simulink model "template_2018b_D"  (R2020a)
settings: Solver=ode1  StartTime=0.0  StopTime=2  FixedStep=1e-6  RelTol=1e-3
undefined symbols (not defined in the file or in its folder): Ion, Lithium
libraries: powerlib x13, powerlib_meascontrol x2, electricdrivelib x1, re_lib x1
settings Model: Creator=ander  LastModifiedBy=delfi
settings DebuggingCC: SFMachineParentedDataDiag=error  ArithmeticOperatorsInVariantConditions=warning
settings SFSimCC: CustomCodeUndefinedFunction=UseInterfaceOnly

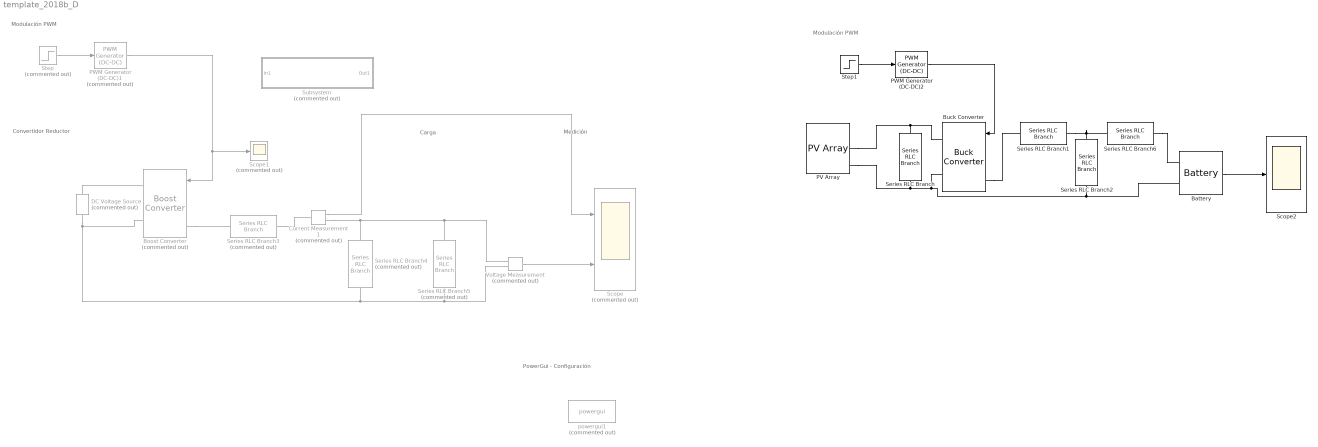
== system template_2018b_D ==
  note: Medición
  note: PowerGui - Configuración
  note: Carga
  note: Convertidor Reductor
  note: Modulación PWM
  note: Modulación PWM
  Battery : electricdrivelib/Extra Sources/Battery  BatType=Lithium-Ion  ShowTempParam=off  ThermalPreset=no  ShowAgeParam=off  NomV=7.2  NomQ=5.4  SOC=100  Batt_Tr=30  PresetModel=on  MaxQ=5.4  MinV=5.4  FullV=8.3807  Dis_rate=2.3478  R=0.013333  Normal_OP=4.8835  expZone="[7.7788      0.2653]"  current=[6.5 13 32.5]  Units=Time  Tci=20  NomT=20  T2=-30  MaxQ2=4.8  FullV2=7.1  Normal_OP2=5.655  expZone2="[6.58           1]"  Rca=0.6  ti=2000  Dp=0  Neq0=0  Tsim=1e6  Ta1=25  Qeol=5.4*0.9  Reol=0.013333*1.2  Char_age=[2.3478, 3]  Dis_age=[2.3478, 10]  N1=1500  N2=10500  N3=1000  N4=1400  Ta2=45  N5=950
  Boost Converter : powerlib/Power Electronics/Boost Converter  Commented=on  ModelType=Switching devices  Ron=1e-3  Rs=1e6  Cs=inf  Vforward=[0,0]  Ron_Diode=1e-3  Rs_Diode=1e6  Cs_Diode=inf  Vf_Diode=1e-3  Rs_CurrentSource=inf
      settings: SourceProductBaseCode=PS
  Buck Converter : powerlib/Power Electronics/Buck Converter  ModelType=Switching devices  Ron=1e-3  Rs=1e6  Cs=inf  Vforward=[0,0]  Ron_Diode=1e-3  Rs_Diode=1e6  Cs_Diode=inf  Vf_Diode=1e-3  Rs_CurrentSource=inf
      settings: SourceProductBaseCode=PS
  Current Measurement1 : powerlib/Measurements/Current Measurement  Commented=on  PhasorSimulation=off  OutputType=Complex  PSBequivalent=0
  DC Voltage Source : powerlib/Electrical Sources/DC Voltage Source  Commented=on  Amplitude=100  Measurements=None
  PV Array : re_lib/Solar/PV Array  Npar=40  Nser=10  PlotType=one module @ 25 deg.C & specified irradiances  S_vec="[ 1000  500  100 ]"  Temp_C_vec="[ 45 25  ]"  ModuleName=User-defined  PlotWhenSelected=off  Pm=30.06  Ncell=60  Voc=21.5  Isc=1.86  Vm=18  Im=1.67  beta_Voc_pc=-0.36  alpha_Isc_pc=0.102  beta_Voc=-0.0774  alpha_Isc=0.0018972  IL=1.8865  I0=6.7437e-11  nI=0.58192  Rsh=136.2109  Rs=0.44647  RobustModel=off  RobustCellTemperature=25  BAL=on  Tc=1e-6  Tfilter=5e-5
  PWM Generator (DC-DC)1 : powerlib_meascontrol/Pulse & Signal Generators/PWM Generator (DC-DC)  Commented=on  Fsw=5000  Ts=0
  PWM Generator (DC-DC)2 : powerlib_meascontrol/Pulse & Signal Generators/PWM Generator (DC-DC)  Fsw=5000  Ts=0
  Scope : Scope  Commented=on  NumInputPorts=2
  Scope1 : Scope  Commented=on
  Scope2 : Scope
  Series RLC Branch : powerlib/Elements/Series RLC Branch  LConnTagsString=__new0  RConnTagsString=__new0  BranchType=C  Resistance=1  Inductance=1e-3  SetiL0=off  InitialCurrent=0  Capacitance=1e-6  Setx0=off  InitialVoltage=0  Measurements=None
  Series RLC Branch1 : powerlib/Elements/Series RLC Branch  LConnTagsString=__new0  RConnTagsString=__new0  BranchType=RL  Resistance=1  Inductance=1e-3  SetiL0=off  InitialCurrent=0  Capacitance=1e-6  Setx0=off  InitialVoltage=0  Measurements=None
  Series RLC Branch2 : powerlib/Elements/Series RLC Branch  LConnTagsString=__new0  RConnTagsString=__new0  BranchType=C  Resistance=1  Inductance=1e-3  SetiL0=off  InitialCurrent=0  Capacitance=1e-6  Setx0=off  InitialVoltage=0  Measurements=None
  Series RLC Branch3 : powerlib/Elements/Series RLC Branch  Commented=on  LConnTagsString=__new0  RConnTagsString=__new0  BranchType=RLC  Resistance=1  Inductance=1e-3  SetiL0=off  InitialCurrent=0  Capacitance=1e-6  Setx0=off  InitialVoltage=0  Measurements=None
  Series RLC Branch4 : powerlib/Elements/Series RLC Branch  Commented=on  LConnTagsString=__new0  RConnTagsString=__new0  BranchType=RLC  Resistance=1  Inductance=1e-3  SetiL0=off  InitialCurrent=0  Capacitance=1e-6  Setx0=off  InitialVoltage=0  Measurements=None
  Series RLC Branch5 : powerlib/Elements/Series RLC Branch  Commented=on  LConnTagsString=__new0  RConnTagsString=__new0  BranchType=RLC  Resistance=1  Inductance=1e-3  SetiL0=off  InitialCurrent=0  Capacitance=1e-6  Setx0=off  InitialVoltage=0  Measurements=None
  Series RLC Branch6 : powerlib/Elements/Series RLC Branch  LConnTagsString=__new0  RConnTagsString=__new0  BranchType=R  Resistance=1  Inductance=1e-3  SetiL0=off  InitialCurrent=0  Capacitance=1e-6  Setx0=off  InitialVoltage=0  Measurements=None
  Step : Step  Commented=on  Before=0.5  After=0.55  SampleTime=0
  Step1 : Step  Before=0.5  After=0.55  SampleTime=0
  Subsystem : Subsystem  Commented=on
  Voltage Measurement : powerlib/Measurements/Voltage Measurement  Commented=on  PhasorSimulation=off  OutputType=Complex  PSBequivalent=0
  powergui1 : powerlib/powergui  Priority=1  Commented=on  SimulationMode=Discrete  SampleTime=50e-6  frequency=60  Iterations=50  frequencyindice=0  Pbase=100e6  ErrMax=1e-4  UnitsV=kV  UnitsW=MW  buscounter=0  FunctionMessages=off  echomessages=off  EnableUseOfTLC=off  CurrentSourceSwitches=off  DisableSnubberDevices=off  DisableRonSwitches=off  DisableVfSwitches=off  DisplayEquations=off  AutomaticDiscreteSolvers=off  SolverType=Tustin/Backward Euler (TBE)  Interpol=off  ExternalGateDelay=off  methode=off  Ts=100  x0status=blocks  SPID=on  SwTol=0  HookPort=off  NonlinearTolerance=1e-4  nMaxIteration=100  ContinueOnMaxIteration=off  RestoreLinks=warning  ResistiveCurrentMeasurement=off  Frange=[0:2:500]  Ylog=off  Xlog=on  ShowGrid=off  save=off  variable=ZData  structure=0  ZoomFFT=off  StartTime=0.0  cycles=1  DisplayStyle=1  fundamental=60  FreqAxis=off  MaxFrequency=1000  frequencyindicesteady=1  RmsSteady=1  display=off
  wires:
  Current Measurement1/1 -> Scope/1
  Voltage Measurement/1 -> Scope/2
  Step/1 -> PWM Generator (DC-DC)1/1
  PWM Generator (DC-DC)1/1 -> Boost Converter/1, Scope1/1
  Step1/1 -> PWM Generator (DC-DC)2/1
  PWM Generator (DC-DC)2/1 -> Buck Converter/1
  Battery/1 -> Scope2/1
  connections:
  Current Measurement1/RConn1 -- Series RLC Branch4/LConn1 -- Series RLC Branch5/LConn1 -- Voltage Measurement/LConn1
  Series RLC Branch3/LConn1 -- Current Measurement1/LConn1
  Series RLC Branch5/RConn1 -- DC Voltage Source/LConn1 -- Boost Converter/RConn2 -- Series RLC Branch4/RConn1 -- Voltage Measurement/LConn2
  Boost Converter/LConn1 -- Series RLC Branch3/RConn1
  DC Voltage Source/RConn1 -- Boost Converter/RConn1
  PV Array/RConn1 -- Series RLC Branch/RConn1 -- Buck Converter/RConn1
  PV Array/RConn2 -- Series RLC Branch/LConn1 -- Battery/LConn2 -- Series RLC Branch2/RConn1 -- Buck Converter/RConn2
  Buck Converter/LConn1 -- Series RLC Branch1/LConn1
  Series RLC Branch1/RConn1 -- Series RLC Branch2/LConn1 -- Series RLC Branch6/LConn1
  Series RLC Branch6/RConn1 -- Battery/LConn1

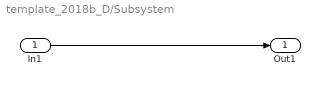
== system template_2018b_D/Subsystem ==
  In1 : Inport
  Out1 : Outport
  wires:
  In1/1 -> Out1/1
